simulink model "resonance_pulse"  (R2022a)
settings: Solver=VariableStepAuto  StartTime=0.0  StopTime=53  MaxStep=1e-3  RelTol=1e-3
libraries: resonance_lib x2
settings Model: Creator=tstef  LastModifiedBy=thomas

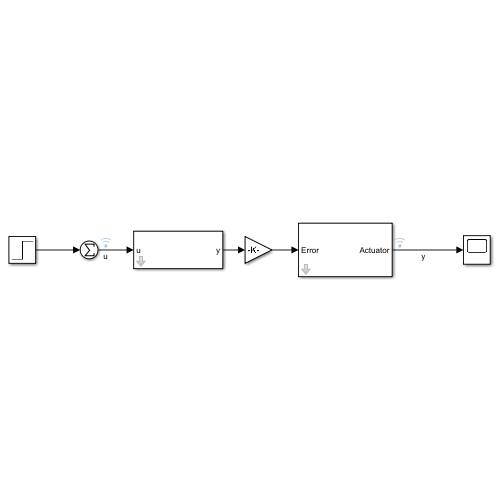
[thumbnail: Simulink's stored preview of the top-level diagram]
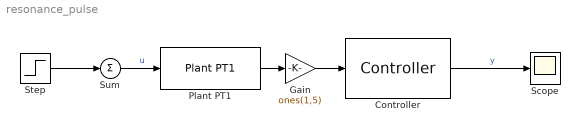
== system resonance_pulse ==
  Controller : resonance_lib/Controller  k_P=2.9  k_I=41  k_R=880  k_Rb=0  T1=0.093  w0=100  zeta=0.05
  Gain : Gain  Gain=ones(1,5)
  Plant PT1 : resonance_lib/Plants/Plant PT1  p=1
  Scope : Scope
  Step : Step  Time=[0.001 0.002 1 51]  After=[1 -1 -0.00002 0.00002]  SampleTime=0
  Sum : Sum  Inputs=+
  wires:
  Controller/1 -> Scope/1  "y"
  Gain/1 -> Controller/1
  Sum/1 -> Plant PT1/1  "u"
  Step/1 -> Sum/1
  Plant PT1/1 -> Gain/1
